simulink model "RLBicycleSimulinkModel"  (R2021a)
settings: Solver=VariableStepAuto  StartTime=0.0  StopTime=200  RelTol=1e-3
model workspace (MAT data in the model file):
  Sig = Simulink.Signal
  Sig.DataType = 'auto'
  Sig.Dimensions = -1
  Sig.DimensionsMode = 'auto'
  Sig.Complexity = 'auto'
  Sig.SampleTime = -1
  Sig.SamplingMode = 'auto'
undefined symbols (not defined in the file or in its folder): chosenMap, startLoc, startOrient
libraries: robotmobilelib x1, rllib x1
settings Model: OrderedModelArguments=off  Creator=The MathWorks, Inc.  LastModifiedBy=guyot
settings SolverCC: AlgebraicLoopSolver=TrustRegion
settings DebuggingCC: SymbolicDimsDataTypeCodeGenerationDiagnostic=none  SFMachineParentedDataDiag=warning

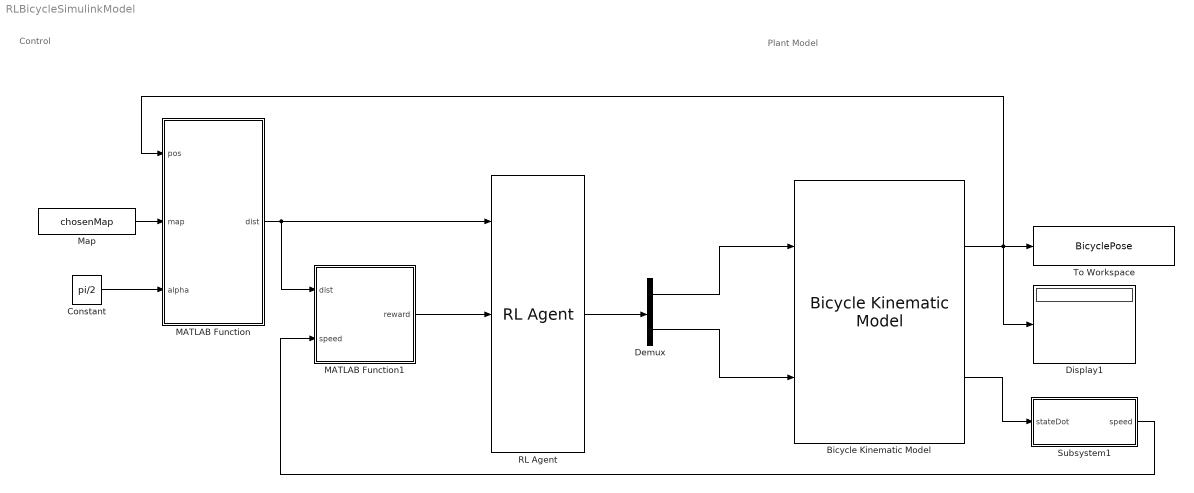
== system RLBicycleSimulinkModel ==
  note: Control
  note: Plant Model
  Bicycle Kinematic Model : robotmobilelib/Bicycle Kinematic Model  VehicleInputs=Vehicle Speed & Heading Angular Velocity  WheelBase=1  VehicleSpeedRange=[-inf, inf]  MaxSteeringAngle=pi/2  InitialState=[startLoc startOrient]  SimulateUsing=Interpreted execution
      settings: SourceProductBaseCode=RO
  Constant : Constant  Value=pi/2
  Demux : Demux  Outputs=2
  Display1 : Display
  MATLAB Function : MATLAB Function  TreatAsAtomicUnit=on
  MATLAB Function1 : MATLAB Function  TreatAsAtomicUnit=on
  Map : Constant  Value=chosenMap
  RL Agent : rllib/RL Agent  Agent=agent  ExternalActionAsInput=off  ProvideCumRwd=off  TreatAsDirectFeedthrough=on
  Subsystem1 : Subsystem
  To Workspace : ToWorkspace  VariableName=BicyclePose  SampleTime=-1
  wires:
  Map/1 -> MATLAB Function/2(map)
  Bicycle Kinematic Model/1 -> To Workspace/1, Display1/1, MATLAB Function/1(pos)
  Demux/2 -> Bicycle Kinematic Model/2
  Demux/1 -> Bicycle Kinematic Model/1
  MATLAB Function/1(dist) -> RL Agent/1, MATLAB Function1/1(dist)
  RL Agent/1 -> Demux/1
  MATLAB Function1/1(reward) -> RL Agent/2
  Constant/1 -> MATLAB Function/3(alpha)
  Bicycle Kinematic Model/2 -> Subsystem1/1(stateDot)
  Subsystem1/1(speed) -> MATLAB Function1/2(speed)

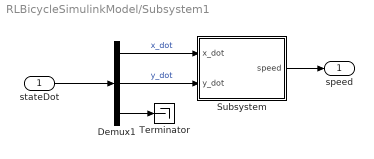
== system RLBicycleSimulinkModel/Subsystem1 ==
  stateDot : Inport
  Demux1 : Demux  Outputs=3
  Subsystem : Subsystem
  Terminator : Terminator
  speed : Outport
  wires:
  Subsystem/1(speed) -> speed/1
  Demux1/3 -> Terminator/1
  Demux1/1 -> Subsystem/1(x_dot)  "x_dot"
  stateDot/1 -> Demux1/1
  Demux1/2 -> Subsystem/2(y_dot)  "y_dot"

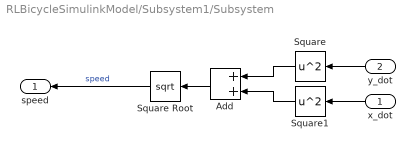
== system RLBicycleSimulinkModel/Subsystem1/Subsystem ==
  x_dot : Inport
  y_dot : Inport  Port=2
  Add : Sum
  Square : Math  Operator=square  SaturateOnIntegerOverflow=on
  Square Root : Sqrt  SaturateOnIntegerOverflow=on
  Square1 : Math  Operator=square  SaturateOnIntegerOverflow=on
  speed : Outport
  wires:
  y_dot/1 -> Square/1
  Square/1 -> Add/1
  Add/1 -> Square Root/1
  Square1/1 -> Add/2
  x_dot/1 -> Square1/1
  Square Root/1 -> speed/1  "speed"

== matlab function RLBicycleSimulinkModel/MATLAB Function ==
  data: pos input; map input; alpha input; dist output
function dist = distMin(pos, map, alpha)
    % Trouve la distance minimale dans un cône devant le véhicule
    % alpha : angle du cône

dist = 0

== matlab function RLBicycleSimulinkModel/MATLAB Function1 ==
  data: dist input; reward output; speed input
function reward = calcRew(dist, speed)
    % Fonction de calcul de recompense
    % coefficients a tuner
    if dist < 0.05
        reward = -100
    elseif dist < 0.1
        reward = 5*dist + speed
    else
        reward = 5*dist + 5*speed
    end
